simulink model "projekat_model_2024b"  (R2024b)
settings: Solver=FixedStepAuto  StartTime=0.0  StopTime=60  FixedStep=Ts  RelTol=1e-3
values from neighbouring files (symbols this model uses):
  sw = 10    [projekat.m]
  sysd_1 = ss(Gd_1)    [projekat.m]
  sysd_2 = ss(Gd_2)    [projekat.m]
  Tf = 1e-2    (= 0.01)    [projekat.m]
  Ts = 1e-3    (= 0.001)    [projekat.m]
  upd = 20    [projekat.m]
undefined symbols (not defined in the file or in its folder): R, tsarrayFcn
settings Model: Creator=Nenad  LastModifiedBy=Nenad
settings ConfigComp: CovBoundaryAbsTol=1.0e-5

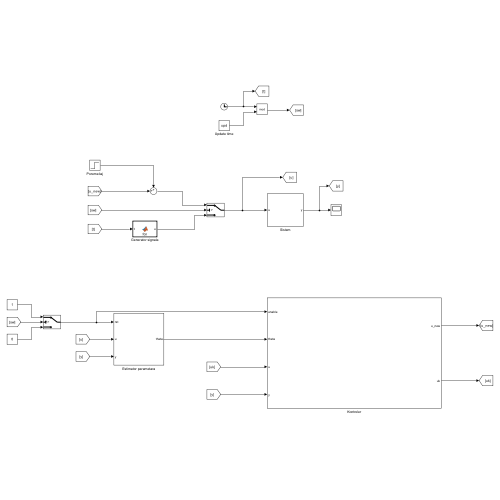
[thumbnail: Simulink's stored preview of the top-level diagram]
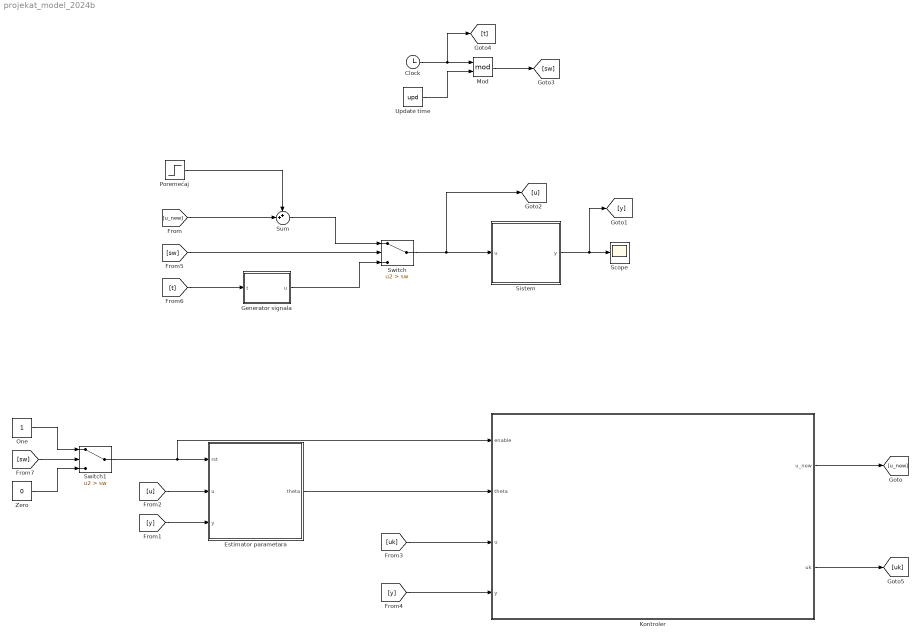
== system projekat_model_2024b ==
  Clock : Clock
  Estimator parametara : Subsystem
  Generator signala : MATLAB Function  TreatAsAtomicUnit=on
  Kontroler : Subsystem
  Mod : Math  Operator=mod
  One : Constant  OutDataTypeStr=Inherit: Inherit via back propagation
  Poremećaj : Step  Time=10  SampleTime=Ts
  Scope : Scope
  Sistem : Subsystem
  Sum : Sum  Inputs=++|
  Switch : Switch  Criteria=u2 > Threshold  Threshold=sw  SaturateOnIntegerOverflow=off  InputSameDT=off
  Switch1 : Switch  Criteria=u2 > Threshold  Threshold=sw  SaturateOnIntegerOverflow=off  InputSameDT=off
  Update time : Constant  Value=upd  OutDataTypeStr=Inherit: Inherit via back propagation
  Zero : Constant  Value=0  OutDataTypeStr=Inherit: Inherit via back propagation  SampleTime=Ts
  wires:
  Generator signala/1(u) -> Switch/3
  [y] -> Estimator parametara/3(y)
  [u] -> Estimator parametara/2(u)
  Estimator parametara/1(theta) -> Kontroler/2(theta)
  [y] -> Kontroler/4("y ")
  Kontroler/1(u_new) -> [u_new]
  Clock/1 -> [t], Mod/1
  Update time/1 -> Mod/2
  Mod/1 -> [sw]
  [sw] -> Switch/2
  [t] -> Generator signala/1(t)
  Switch1/1 -> Kontroler/1(enable), Estimator parametara/1(rst)
  [sw] -> Switch1/2
  One/1 -> Switch1/1
  Zero/1 -> Switch1/3
  Sistem/1(y) -> [y], Scope/1
  Switch/1 -> [u], Sistem/1(u)
  [u_new] -> Sum/2
  Sum/1 -> Switch/1
  Poremećaj/1 -> Sum/1
  [uk] -> Kontroler/3(u)
  Kontroler/2(uk) -> [uk]

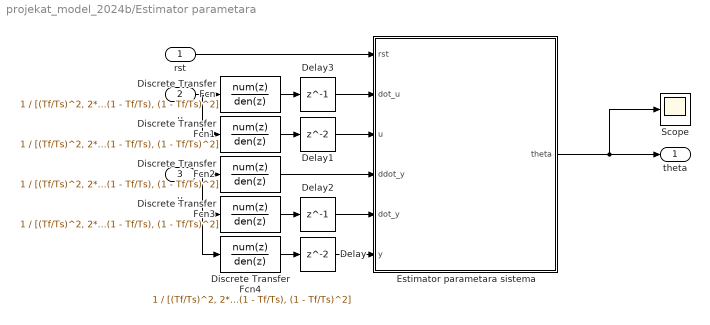
== system projekat_model_2024b/Estimator parametara ==
  rst : Inport
  u : Inport  Port=2
  y : Inport  Port=3
  Delay : Delay
  Delay1 : Delay
  Delay2 : Delay  DelayLength=1
  Delay3 : Delay  DelayLength=1
  Discrete Transfer Fcn{,1..4} (5 alike) : DiscreteTransferFcn  Numerator=1  Denominator=[(Tf/Ts)^2, 2*(Tf/Ts)*(1 - Tf/Ts), (1 - Tf/Ts)^2]
  Estimator parametara sistema : MATLAB Function  TreatAsAtomicUnit=on
  Scope : Scope
  theta : Outport
  wires:
  Estimator parametara sistema/1(theta) -> Scope/1, theta/1
  Delay/1 -> Estimator parametara sistema/6(y)
  Delay1/1 -> Estimator parametara sistema/3(u)
  Delay3/1 -> Estimator parametara sistema/2(dot_u)
  u/1 -> Discrete Transfer Fcn1/1, Discrete Transfer Fcn/1
  Discrete Transfer Fcn/1 -> Delay3/1
  Discrete Transfer Fcn1/1 -> Delay1/1
  y/1 -> Discrete Transfer Fcn3/1, Discrete Transfer Fcn4/1, Discrete Transfer Fcn2/1
  Discrete Transfer Fcn2/1 -> Estimator parametara sistema/4(ddot_y)
  Discrete Transfer Fcn3/1 -> Delay2/1
  Delay2/1 -> Estimator parametara sistema/5(dot_y)
  Discrete Transfer Fcn4/1 -> Delay/1
  rst/1 -> Estimator parametara sistema/1(rst)

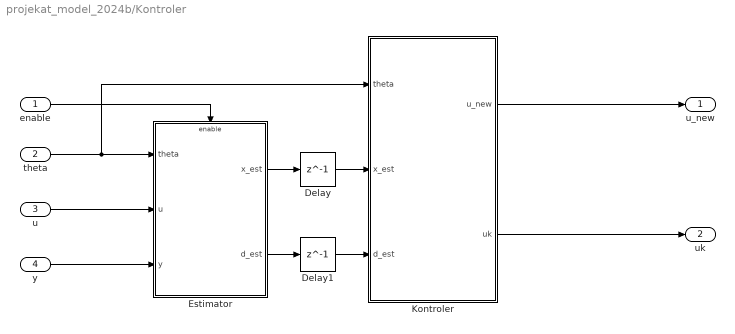
== system projekat_model_2024b/Kontroler ==
  enable : Inport
  theta : Inport  Port=2
  u : Inport  Port=3
  "y " : Inport  Port=4
  Delay : Delay  DelayLength=1
  Delay1 : Delay  DelayLength=1
  Estimator : Subsystem
  Kontroler : Subsystem
  u_new : Outport
  uk : Outport  Port=2
  wires:
  enable/1 -> Estimator/Enable
  theta/1 -> Kontroler/1(theta), Estimator/1(theta)
  "y "/1 -> Estimator/3("y ")
  u/1 -> Estimator/2(u)
  Kontroler/1(u_new) -> u_new/1
  Estimator/1(x_est) -> Delay/1
  Delay/1 -> Kontroler/2(x_est)
  Delay1/1 -> Kontroler/3(d_est)
  Estimator/2(d_est) -> Delay1/1
  Kontroler/2(uk) -> uk/1

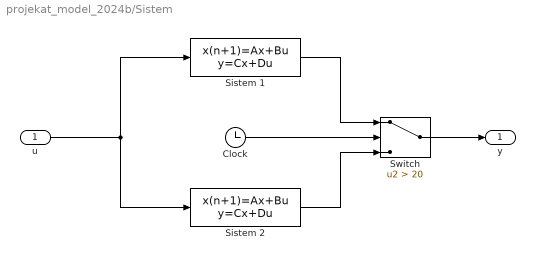
== system projekat_model_2024b/Sistem ==
  u : Inport
  Clock : Clock
  Sistem 1 : DiscreteStateSpace  A=sysd_1.A  B=sysd_1.B  C=sysd_1.C  D=sysd_1.D  SampleTime=Ts
  Sistem 2 : DiscreteStateSpace  A=sysd_2.A  B=sysd_2.B  C=sysd_2.C  D=sysd_2.D  SampleTime=Ts
  Switch : Switch  Criteria=u2 > Threshold  Threshold=20  SaturateOnIntegerOverflow=off  InputSameDT=off
  y : Outport
  wires:
  u/1 -> Sistem 2/1, Sistem 1/1
  Switch/1 -> y/1
  Sistem 1/1 -> Switch/1
  Sistem 2/1 -> Switch/3
  Clock/1 -> Switch/2

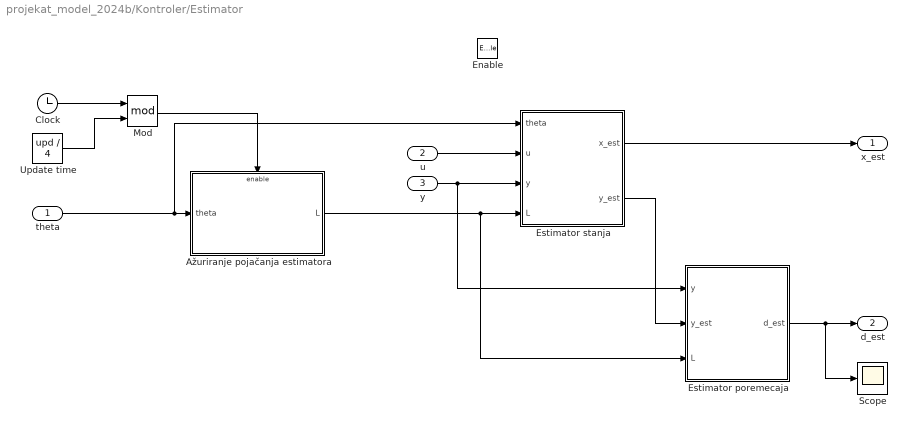
== system projekat_model_2024b/Kontroler/Estimator ==
  theta : Inport
  u : Inport  Port=2
  "y " : Inport  Port=3
  Enable : EnablePort
  Ažuriranje pojačanja estimatora : Subsystem
  Clock : Clock
  Estimator poremecaja : MATLAB Function  TreatAsAtomicUnit=on
  Estimator stanja : MATLAB Function  TreatAsAtomicUnit=on
  Mod : Math  Operator=mod
  Scope : Scope
  Update time : Constant  Value=upd / 4  OutDataTypeStr=Inherit: Inherit via back propagation
  x_est : Outport
  d_est : Outport  Port=2
  wires:
  Estimator stanja/1(x_est) -> x_est/1
  "y "/1 -> Estimator poremecaja/1(y), Estimator stanja/3(y)
  u/1 -> Estimator stanja/2(u)
  Clock/1 -> Mod/1
  Update time/1 -> Mod/2
  Mod/1 -> Ažuriranje pojačanja estimatora/Enable
  theta/1 -> Estimator stanja/1(theta), Ažuriranje pojačanja estimatora/1(theta)
  Ažuriranje pojačanja estimatora/1(L) -> Estimator poremecaja/3(L), Estimator stanja/4(L)
  Estimator poremecaja/1(d_est) -> d_est/1, Scope/1
  Estimator stanja/2(y_est) -> Estimator poremecaja/2(y_est)

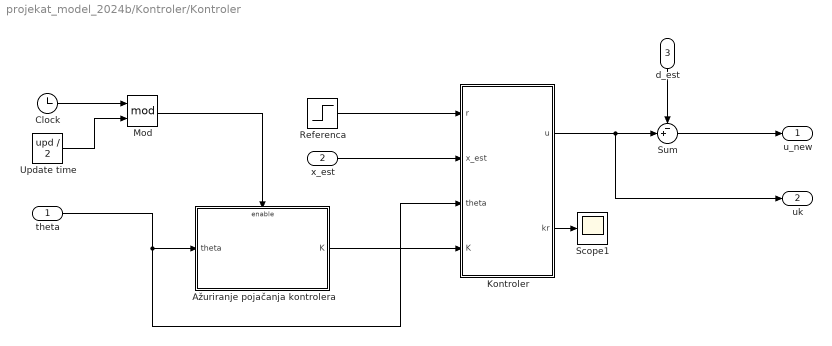
== system projekat_model_2024b/Kontroler/Kontroler ==
  theta : Inport
  x_est : Inport  Port=2
  d_est : Inport  Port=3
  Ažuriranje pojačanja kontrolera : Subsystem
  Clock : Clock
  Kontroler : MATLAB Function  TreatAsAtomicUnit=on
  Mod : Math  Operator=mod
  Referenca : Step  Time=0  After=R  SampleTime=tsarrayFcn
  Scope1 : Scope
  Sum : Sum  Inputs=-+|
  Update time : Constant  Value=upd / 2  OutDataTypeStr=Inherit: Inherit via back propagation  SampleTime=Ts
  u_new : Outport
  uk : Outport  Port=2
  wires:
  x_est/1 -> Kontroler/2(x_est)
  Update time/1 -> Mod/2
  Clock/1 -> Mod/1
  Mod/1 -> Ažuriranje pojačanja kontrolera/Enable
  theta/1 -> Kontroler/3(theta), Ažuriranje pojačanja kontrolera/1(theta)
  Ažuriranje pojačanja kontrolera/1(K) -> Kontroler/4(K)
  Kontroler/2(kr) -> Scope1/1
  Kontroler/1(u) -> Sum/2, uk/1
  d_est/1 -> Sum/1
  Referenca/1 -> Kontroler/1(r)
  Sum/1 -> u_new/1

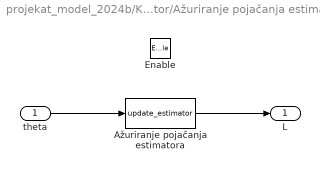
== system projekat_model_2024b/Kontroler/Estimator/Ažuriranje pojačanja estimatora ==
  theta : Inport
  Enable : EnablePort
  Ažuriranje pojačanja estimatora : MATLABFcn  MATLABFcn=update_estimator  OutputDimensions=[3, 1]  Output1D=off
  L : Outport
  wires:
  theta/1 -> Ažuriranje pojačanja estimatora/1
  Ažuriranje pojačanja estimatora/1 -> L/1

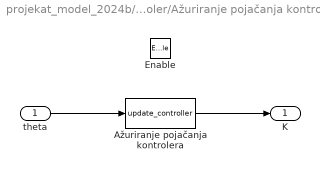
== system projekat_model_2024b/Kontroler/Kontroler/Ažuriranje pojačanja kontrolera ==
  theta : Inport
  Enable : EnablePort
  Ažuriranje pojačanja kontrolera : MATLABFcn  MATLABFcn=update_controller  OutputDimensions=[1, 2]  Output1D=off
  K : Outport
  wires:
  theta/1 -> Ažuriranje pojačanja kontrolera/1
  Ažuriranje pojačanja kontrolera/1 -> K/1

== matlab function projekat_model_2024b/Estimator parametara/Estimator parametara sistema ==
  settings: updateMethod=DISCRETE  sampleTime=Ts
  data: rst input; dot_u input; u input; ddot_y input; dot_y input; theta output; y input
function theta = fcn(rst, dot_u, u, ddot_y, dot_y, y)
    persistent P;
    persistent Theta;
    lambda = 0.999;
    
    phi = [-dot_y; -y; dot_u; u];
    eta = ddot_y;
    
    if isempty(Theta)
        Theta = zeros(length(phi), 1);
    end

    if isempty(P) || rst == 1
        P = 10e8 * eye(length(phi), length(phi));
    end

    if rst == 1
        theta = Theta;
        return
    end

    P = 1 / lambda * (P - (P * (phi * phi') * P) / (lambda + phi' * P * phi));
    
    Theta = Theta + P * phi * (eta - phi' * Theta);
    theta = Theta;
end

== matlab function projekat_model_2024b/Generator signala ==
  data: t input; u output
function u = fcn(t)
    u = 1;
    fmax = 50;

    for f = 1:fmax
        u = u + sin(2 * pi * f * t);
    end
end

== matlab function projekat_model_2024b/Kontroler/Estimator/Estimator stanja ==
  settings: updateMethod=DISCRETE  sampleTime=Ts
  data: theta input; u input; x_est output; y input; L input; y_est output
function [x_est, y_est] = fcn(theta, u, y, L)
   persistent x

   if isempty(x)
       x = [0; 0];
   end

   a1 = theta(1);
   a0 = theta(2);
   b1 = theta(3);
   b0 = theta(4);

   A = [0, 1; -a0, -a1];
   B = [0; 1];
   C = [b0, b1];

   x_est = x;
   y_est = C * x;
   Lx = L(1:2);

   x_next = (A - Lx * C) * x + [B, Lx] * [u; y];
   x = x_next;
end

== matlab function projekat_model_2024b/Kontroler/Kontroler/Kontroler ==
  settings: updateMethod=DISCRETE  sampleTime=Ts
  data: r input; x_est input; theta input; u output; K input; kr output
function [u, kr] = fcn(r, x_est, theta, K)
    a1 = theta(1);
    a0 = theta(2);
    b1 = theta(3);
    b0 = theta(4);

    k1 = K(1);
    k2 = K(2);

    kr = (1 + a1 + a0 + k1 + k2) / (b1 + b0);
    u = -K * x_est + kr * r;
end

== matlab function projekat_model_2024b/Kontroler/Estimator/Estimator poremecaja ==
  settings: updateMethod=DISCRETE  sampleTime=Ts
  data: y input; y_est input; d_est output; L input
function d_est = fcn(y, y_est, L)
   persistent w

   if isempty(w)
       w = 0;
   end

   Aw = 1;
   Lw = L(3);

   w_next = Aw * w + Lw * (y - y_est);
   d_est = w_next;
   
   w = w_next;
end
